simulink model "projectminor"  (R2024b)
settings: Solver=VariableStepAuto  StartTime=0.0  StopTime=50  RelTol=1e-3
model workspace (MAT data in the model file):
  Ts = 0.1
libraries: mpcadaslib x1

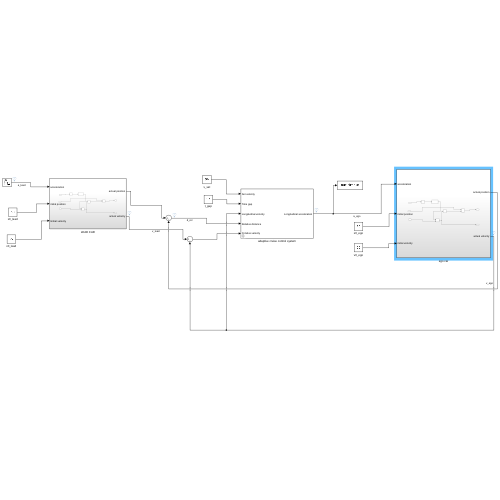
[thumbnail: Simulink's stored preview of the top-level diagram]
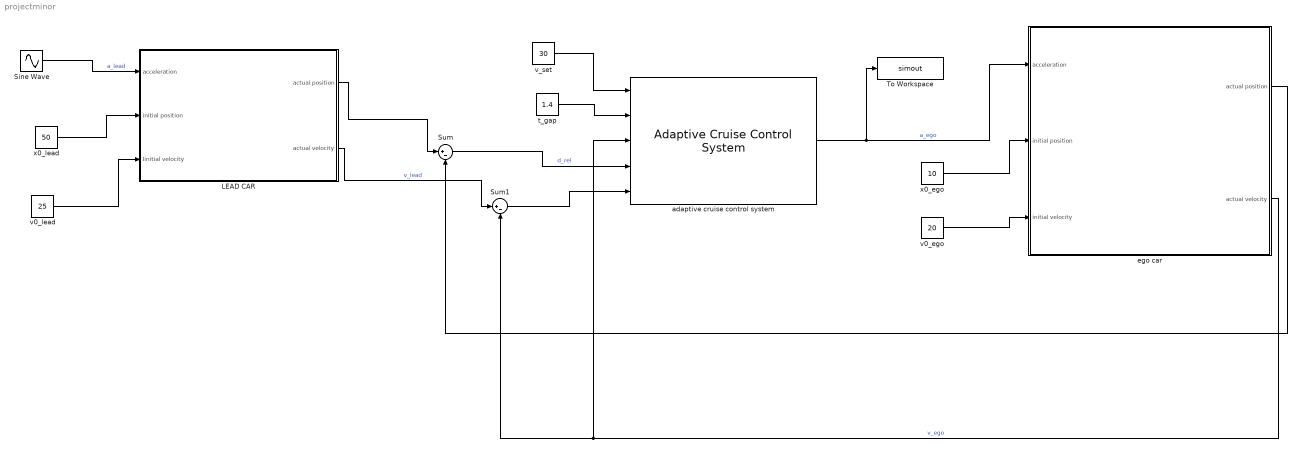
== system projectminor ==
  LEAD CAR : Subsystem
  Sine Wave : Sin  Amplitude=0.6  Frequency=0.2  SampleTime=Ts
  Sum : Sum  Inputs=|+-
  Sum1 : Sum  Inputs=|+-
  To Workspace : ToWorkspace  VariableName=simout  SaveFormat=Timeseries  SampleTime=-1
  adaptive cruise control system : mpcadaslib/Adaptive Cruise Control System  EgoModel=tf(1,[0.5,1,0])  InitialEgoVelocity=20  DefaultSpacing=10  MaxVelocity=50  MinAcceleration=-3  amin_ext=off  MaxAcceleration=2  amax_ext=off  Ts=0.1  PredictionHorizon=30  ControllerBehavior=0.5  suboptimal=off  maxiter=10  datatypeopt=double  optmode=off  trackmode=off
      settings: LibrarySourceBlock=mpclib/Automated Driving/Adaptive Cruise Control System
  ego car : Subsystem
  t_gap : Constant  Value=1.4  SampleTime=Ts
  v0_ego : Constant  Value=20  SampleTime=Ts
  v0_lead : Constant  Value=25  SampleTime=Ts
  v_set : Constant  Value=30  SampleTime=Ts
  x0_ego : Constant  Value=10  SampleTime=Ts
  x0_lead : Constant  Value=50  SampleTime=Ts
  wires:
  Sine Wave/1 -> LEAD CAR/1(acceleration)  "a_lead"
  x0_lead/1 -> LEAD CAR/2(initial position)
  v0_lead/1 -> LEAD CAR/3(Iinitial velocity)
  LEAD CAR/1(actual position) -> Sum/1
  LEAD CAR/2(actual velocity) -> Sum1/1  "v_lead"
  adaptive cruise control system/1 -> To Workspace/1, ego car/1(acceleration)  "a_ego"
  x0_ego/1 -> ego car/2(initial position)
  v0_ego/1 -> ego car/3(initial velocity)
  ego car/1(actual position) -> Sum/2
  ego car/2(actual velocity) -> adaptive cruise control system/3, Sum1/2  "v_ego"
  v_set/1 -> adaptive cruise control system/1
  t_gap/1 -> adaptive cruise control system/2
  Sum/1 -> adaptive cruise control system/4  "d_rel"
  Sum1/1 -> adaptive cruise control system/5

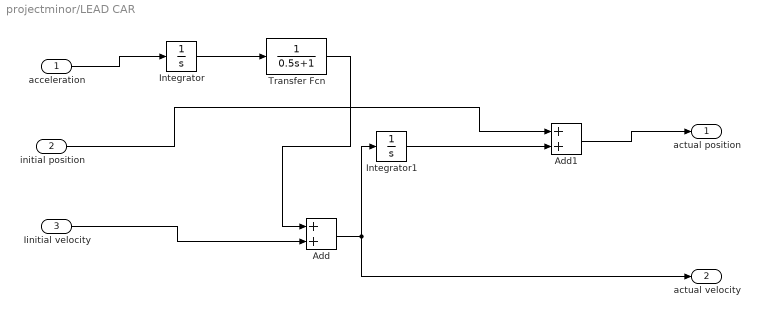
== system projectminor/LEAD CAR ==
  acceleration : Inport
  initial position : Inport  Port=2
  Iinitial velocity : Inport  Port=3
  Add : Sum
  Add1 : Sum
  Integrator : Integrator
  Integrator1 : Integrator
  Transfer Fcn : TransferFcn  Denominator=[0.5 1]
  actual position : Outport
  actual velocity : Outport  Port=2
  wires:
  Integrator/1 -> Transfer Fcn/1
  Transfer Fcn/1 -> Add/1
  Integrator1/1 -> Add1/2
  Add/1 -> actual velocity/1, Integrator1/1
  Add1/1 -> actual position/1
  Iinitial velocity/1 -> Add/2
  acceleration/1 -> Integrator/1
  initial position/1 -> Add1/1

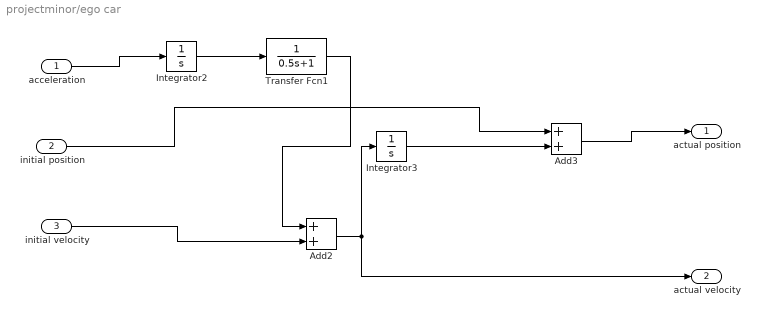
== system projectminor/ego car ==
  acceleration : Inport
  initial position : Inport  Port=2
  initial velocity : Inport  Port=3
  Add2 : Sum
  Add3 : Sum
  Integrator2 : Integrator
  Integrator3 : Integrator
  Transfer Fcn1 : TransferFcn  Denominator=[0.5 1]
  actual position : Outport
  actual velocity : Outport  Port=2
  wires:
  Integrator2/1 -> Transfer Fcn1/1
  Add3/1 -> actual position/1
  Transfer Fcn1/1 -> Add2/1
  acceleration/1 -> Integrator2/1
  Add2/1 -> actual velocity/1, Integrator3/1
  Integrator3/1 -> Add3/2
  initial velocity/1 -> Add2/2
  initial position/1 -> Add3/1
